simulink model "Factorial__Forloop"  (R2021a)
settings: Solver=VariableStepAuto  StartTime=0.0  StopTime=10.0  RelTol=1e-3
settings Model: Creator=Nour  LastModifiedBy=Nour

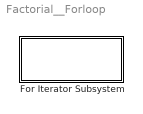
== system Factorial__Forloop ==
  For Iterator Subsystem : Subsystem  TreatAsAtomicUnit=on

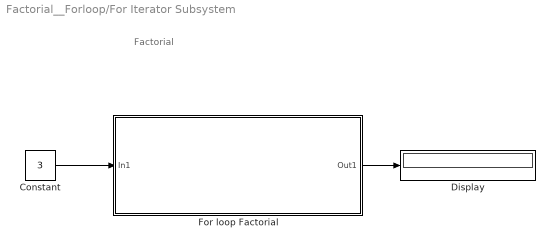
== system Factorial__Forloop/For Iterator Subsystem ==
  note: Factorial
  Constant : Constant  Value=3  OutDataTypeStr=uint32  SampleTime=-1
  Display : Display
  For loop Factorial : Subsystem
  wires:
  Constant/1 -> For loop Factorial/1(In1)
  For loop Factorial/1(Out1) -> Display/1

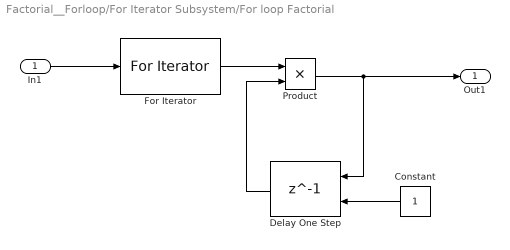
== system Factorial__Forloop/For Iterator Subsystem/For loop Factorial ==
  In1 : Inport
  Constant : Constant  OutDataTypeStr=uint32  SampleTime=-1
  Delay One Step : Delay  DelayLength=1  InitialConditionSource=Input port
      settings: InputPortMap=u0,p4
  For Iterator : ForIterator  IterationSource=external  IterationVariableDataType=uint32
  Product : Product  OutDataTypeStr=uint32
  Out1 : Outport
  wires:
  For Iterator/1 -> Product/1
  Delay One Step/1 -> Product/2
  Constant/1 -> Delay One Step/2
  In1/1 -> For Iterator/1
  Product/1 -> Out1/1, Delay One Step/1
